simulink model "sm_vehicle_2axle_heave_roll_mu"  (R2025b)
settings: Solver=ode23t  StartTime=0.0  StopTime=14.2  MaxStep=0.2  RelTol=1e-3  AbsTol=1e-3  EnableMultiTasking=on
PostLoadFcn:
  | sm_vehicle_2axle_heave_roll_param
  | sm_vehicle_2axle_heave_roll_scene
  | sm_vehicle_2axle_heave_roll_config_maneuver(bdroot,VehicleData,'plateau');
  | set_param([bdroot '/Vehicle'],'popup_surface_conditions','Checker Right');
StartFcn:
  | tic
StopFcn:
  | Elapsed_Sim_Time = toc;
undefined symbols (not defined in the file): brake_trqTs, Disc, FL, FR, Hydraulic, InitVehicle, Mode, RL, RR, SceneData, valve_maxA, valve_maxO, VehicleData, X, Y, Z
libraries: fl_lib x92, sm_lib x43, nesl_utility x40, sm_vehicle_utilities_lib x21, sdlc_lib x8, SimscapeFluids_lib x8, simulink x2, simulink_extras x1
(part 1 of 5)
CloseFcn:
  | try,close(h1_sm_vehicle_2axle_heave_roll),end
  | clear h1_sm_vehicle_2axle_heave_roll
  | try,close(h2_sm_vehicle_2axle_heave_roll),end
  | clear h2_sm_vehicle_2axle_heave_roll
  | try,close(h3_sm_vehicle_2axle_heave_roll),end
  | clear h3_sm_vehicle_2axle_heave_roll
  | 
  | 
  | clear simlog_sm_vehicle_2axle_heave_roll
  | clear logsout_sm_vehicle_2axle_heave_roll
Description:
  | Vehicle Dynamics, 14 DOF Model, Varying Surface Friction
  | 
  | Copyright 2022-2024 The MathWorks, Inc.
settings Model: Creator=smiller  LastModifiedBy=bob
settings SolverCC: AutoScaleAbsTol=off  AlgebraicLoopSolver=TrustRegion
settings DataIOCC: SaveFormat=Array  SaveOutput=off  ReturnWorkspaceOutputs=off  SignalLoggingName=logsout_sm_vehicle_2axle_heave_roll_mu  OutputTimes=[0:0.01:10]
settings OptimizationCC: ReuseModelBlockBuffer=off  ExpressionDepthLimit=2147483647.0  LifeSpan=inf
settings DebuggingCC: UnderspecifiedInitializationDetection=Classic  MergeDetectMultiDrivingBlocksExec=none  SolverPrmCheckMsg=warning  UnconnectedInputMsg=warning  UnconnectedOutputMsg=warning  UnconnectedLineMsg=warning  StateNameClashWarn=warning  PregeneratedLibrarySubsystemCodeDiagnostic=none  SFUnexpectedBacktrackingDiag=warning  SFNoUnconditionalDefaultTransitionDiag=warning  SFExecutionAtInitializationDiag=none  ArithmeticOperatorsInVariantConditions=warning
settings HardwareCC: ProdBitPerPointer=32.0  ProdBitPerSizeT=32.0  ProdBitPerPtrDiffT=32.0  ProdLargestAtomicFloat=None  ProdIntDivRoundTo=Undefined  ProdEndianess=Unspecified  ProdWordSize=32.0  ProdHWDeviceType=32-bit Generic
settings ModelReferenceCC: EnableRefExpFcnMdlSchedulingChecks=on  PropagateSignalLabelsOutOfModel=off
settings SFSimCC: SimUseLocalCustomCode=off  CustomCodeUndefinedFunction=UseInterfaceOnly
settings RTWCC: RTWUseLocalCustomCode=off  GPUComputeCapability=3.5  DLArmComputeVersion=19.05
settings CodeAppCC: StateflowObjectComments=on
settings GRTTargetCC: TargetLangStandard=C89/C90 (ANSI)
settings ConfigComp: CovMetricSettings=dw  CovSaveCumulativeToWorkspaceVar=on  CovSaveSingleToWorkspaceVar=on  CovExternalEMLEnable=off
settings SimscapeCC: SimscapeNormalizeSystem=off  SimscapeLogType=all  SimscapeLogToSDI=on  SimscapeLogName=simlog_sm_vehicle_2axle_heave_roll_mu  SimscapeLogLimitData=off  SimscapeLogDataHistory=50000.0
settings ConfigurationSet: Description=SimMechanics 2G
settings DiagnosticsConfigSet: SimMechanicsUnconnectedFramePorts=none  SimMechanicsConflictingReferenceFrames=none
settings ExplorerConfigSet: InternalSimMechanicsExplorerSettings="<ExplorerConfiguration><canonicalview>default</canonicalview><AnimationSetting><BasePlaybackSpeed>1.0</BasePlaybackSpeed><PlaybackSpeedFactor>2.0</PlaybackSpeedFactor></AnimationSetting><TilePanel><TileInfo><Tiles Columns=\"2\" Count=\"3\" Rows=\"2\"><Column Weight=\"0.6147\"/><Column Weight=\"0.3853\"/><Row Weight=\"0.3693\"/><Row Weight=\"0.6307\"/><Tile Height=\"1\" Width=\"1\" X=\"0\" Y=\"0\"/><Tile Height=\"1\" Width=\"1\" X=\"0\" Y=\"1\"/><Tile Height=\"2\" Width=\"1\" X=\"1\" Y=\"0\"/></Tiles></TileInfo><SceneInfo><SceneViewer><BGColor><R>1</R><G>1</G><B>1</B></BGColor><Camera><DoPerspective>on</DoPerspective><Position><X>-1.49999999999999911</X><Y>1.54074395550978868e-32</Y><Z>10.6999999999999993</Z></Position><Center><X>-1.49999999999999911</X><Y>1.54074395550978868e-32</Y><Z>9.69999999999999929</Z></Center><Up><X>0</X><Y>1</Y><Z>0</Z></Up><ViewLimDist>1</ViewLimDist><YLim>0.466307658154998583</YLim><XLim>1.34838716914770518</XLim></Camera></SceneViewer><SceneViewer><BGColor><R>1</R><G>1</G><B>1</B></BGColor><Camera><DoPerspective>on</DoPerspective><Position><X>2.34000000000000163</X><Y>-3.20000000000000151</Y><Z>1.80000000000000004</Z></Position><Center><X>1.58973091910295716</X><Y>-2.57477576591913149</Y><Z>1.58507916953470085</Z></Center><Up><X>-0.16510675539218278</X><Y>0.137588962826818928</Y><Z>0.976631474319820447</Z></Up><ViewLimDist>1</ViewLimDist><YLim>0.466307658154998583</YLim><XLim>0.779836453951521791</XLim></Camera></SceneViewer><SceneViewer><BGColor><R>1</R><G>1</G><B>1</B></BGColor><Camera><DoPerspective>on</DoPerspective><Position><X>-6.5</X><Y>3.46944695195361419e-16</Y><Z>1.79999999999999982</Z></Position><Center><X>-5.52335553329491002</X><Y>3.46944695195361419e-16</Y><Z>1.58513821732488003</Z></Center><Up><X>0.214861782675119795</X><Y>-1.71056941445900502e-49</Y><Z>0.976644466705089975</Z></Up><ViewLimDist>1</ViewLimDist><YLim>0.466307658154998583</YLim><XLim>0.303969645724483983</XLim></Camera></SceneViewer></SceneInfo></TilePanel><MechEditorPanel><Cameras><Camera><Id>Camera1</Id><Value><Name>Track FixO FR</Name><NativeCamera><PositionTrackingFeature>Vehicle.Camera_Frames.Frame_FixO_FR.R</PositionTrackingFeature><CenterTrackingFeature>Vehicle.Camera_Frames.Frame_FixO_FR.R</CenterTrackingFeature><UpVectorTrackingFeature>Vehicle.Camera_Frames.Frame_FixO_FR.R</UpVectorTrackingFeature><CenterTrackingOrigin>off</CenterTrackingOrigin><CenterTrackingDirection>+X</CenterTrackingDirection><UpVectorTrackingDirection>+Z</UpVectorTrackingDirection></NativeCamera></Value></Camera><Camera><Id>Camera2</Id><Value><Name>Track FixO Right</Name><NativeCamera><PositionTrackingFeature>Vehicle.Camera_Frames.Frame_FixO_Right.R</PositionTrackingFeature><CenterTrackingFeature>Vehicle.Camera_Frames.Frame_FixO_Right.R</CenterTrackingFeature><UpVectorTrackingFeature>Vehicle.Camera_Frames.Frame_FixO_Right.R</UpVectorTrackingFeature><CenterTrackingOrigin>off</CenterTrackingOrigin><CenterTrackingDirection>+X</CenterTrackingDirection><UpVectorTrackingDirection>+Z</UpVectorTrackingDirection></NativeCamera></Value></Camera><Camera><Id>Camera3</Id><Value><Name>Track FixO RR</Name><NativeCamera><PositionTrackingFeature>Vehicle.Camera_Frames.Frame_FixO_RR.R</PositionTrackingFeature><CenterTrackingFeature>Vehicle.Camera_Frames.Frame_FixO_RR.R</CenterTrackingFeature><UpVectorTrackingFeature>Vehicle.Camera_Frames.Frame_FixO_RR.R</UpVectorTrackingFeature><CenterTrackingOrigin>off</CenterTrackingOrigin><CenterTrackingDirection>+X</CenterTrackingDirection><UpVectorTrackingDirection>+Z</UpVectorTrackingDirection></NativeCamera></Value></Camera><Camera><Id>Camera4</Id><Value><Name>Track FixO RL</Name><NativeCamera><PositionTrackingFeature>Vehicle.Camera_Frames.Frame_FixO_RL.R</PositionTrackingFeature><CenterTrackingFeature>Vehicle.Camera_Frames.Frame_FixO_RL.R</CenterTrackingFeature><UpVectorTrackingFeature>Vehicle.Camera_Frames.Frame_FixO_RL.R</UpVectorTrackingFeature><CenterTrackingOrigin>off</CenterTrackingOrigin><CenterTrackingDirection>+X</CenterTrackingDirection><UpVectorTrackingDirection>+Z</UpVectorTrackingDirection></NativeCamera></Value></Camera><Camera><Id>Camera5</Id><Value><Name>Track FixO Left</Name><NativeCamera><PositionTrackingFeature>Vehicle.Camera_Frames.Frame_FixO_Left.R</PositionTrackingFeature><CenterTrackingFeature>Vehicle.Camera_Frames.Frame_FixO_Left.R</CenterTrackingFeature><UpVectorTrackingFeature>Vehicle.Camera_Frames.Frame_FixO_Left.R</UpVectorTrackingFeature><CenterTrackingOrigin>off</CenterTrackingOrigin><CenterTrackingDirection>+X</CenterTrackingDirection><UpVectorTrackingDirection>+Z</UpVectorTrackingDirection></NativeCamera></Value></Camera><Camera><Id>Camera6</Id><Value><Name>Track FixO FL</Name><NativeCamera><PositionTrackingFeature>Vehicle.Camera_Frames.Frame_FixO_FL.R</PositionTrackingFeature><CenterTrackingFeature>Vehicle.Camera_Frames.Frame_FixO_FL.R</CenterTrackingFeature><UpVectorTrackingFeature>Vehicle.Camera_Frames.Frame_FixO_FL.R</UpVectorTrackingFeature><CenterTrackingOrigin>off</CenterTrackingOrigin><CenterTrackingDirection>+X</CenterTrackingDirection><UpVectorTrackingDirection>+Z</UpVectorTrackingDirection></NativeCamera></Value></Camera><Camera><Id>Camera7</Id><Value><Name>Track FixO Top</Name><NativeCamera><PositionTrackingFeature>Vehicle.Camera_Frames.Frame_FixO_Top.R</PositionTrackingFeature><CenterTrackingFeature>Vehicle.Camera_Frames.Frame_FixO_Top.R</CenterTrackingFeature><UpVectorTrackingFeature>Vehicle.Camera_Frames.Frame_FixO_Top.R</UpVectorTrackingFeature><CenterTrackingOrigin>off</CenterTrackingOrigin><CenterTrackingDirection>+X</CenterTrackingDirection><UpVectorTrackingDirection>+Z</UpVectorTrackingDirection></NativeCamera></Value></Camera><Camera><Id>Camera8</Id><Value><Name>Track FixO Front</Name><NativeCamera><PositionTrackingFeature>Vehicle.Camera_Frames.Frame_FixO_Front.R</PositionTrackingFeature><CenterTrackingFeature>Vehicle.Camera_Frames.Frame_FixO_Front.R</CenterTrackingFeature><UpVectorTrackingFeature>Vehicle.Camera_Frames.Frame_FixO_Front.R</UpVectorTrackingFeature><CenterTrackingOrigin>off</CenterTrackingOrigin><CenterTrackingDirection>+X</CenterTrackingDirection><UpVectorTrackingDirection>+Z</UpVectorTrackingDirection></NativeCamera></Value></Camera><Camera><Id>Camera9</Id><Value><Name>Track FixO Rear</Name><NativeCamera><PositionTrackingFeature>Vehicle.Camera_Frames.Frame_FixO_Rear.R</PositionTrackingFeature><CenterTrackingFeature>Vehicle.Camera_Frames.Frame_FixO_Rear.R</CenterTrackingFeature><UpVectorTrackingFeature>Vehicle.Camera_Frames.Frame_FixO_Rear.R</UpVectorTrackingFeature><CenterTrackingOrigin>off</CenterTrackingOrigin><CenterTrackingDirection>+X</CenterTrackingDirection><UpVectorTrackingDirection>+Z</UpVectorTrackingDirection></NativeCamera></Value></Camera><Camera><Id>Camera10</Id><Value><Name>Track FR</Name><NativeCamera><PositionTrackingFeature>Vehicle.Camera_Frames.Frame_FR.R</PositionTrackingFeature><CenterTrackingFeature>Vehicle.Camera_Frames.Frame_FR.R</CenterTrackingFeature><UpVectorTrackingFeature>Vehicle.Camera_Frames.Frame_FR.R</UpVectorTrackingFeature><CenterTrackingOrigin>off</CenterTrackingOrigin><CenterTrackingDirection>+X</CenterTrackingDirection><UpVectorTrackingDirection>+Z</UpVectorTrackingDirection></NativeCamera></Value></Camera><Camera><Id>Camera11</Id><Value><Name>Track Right</Name><NativeCamera><PositionTrackingFeature>Vehicle.Camera_Frames.Frame_Right.R</PositionTrackingFeature><CenterTrackingFeature>Vehicle.Camera_Frames.Frame_Right.R</CenterTrackingFeature><UpVectorTrackingFeature>Vehicle.Camera_Frames.Frame_Right.R</UpVectorTrackingFeature><CenterTrackingOrigin>off</CenterTrackingOrigin><CenterTrackingDirection>+X</CenterTrackingDirection><UpVectorTrackingDirection>+Z</UpVectorTrackingDirection></NativeCamera></Value></Camera><Camera><Id>Camera12</Id><Value><Name>Track RR</Name><NativeCamera><PositionTrackingFeature>Vehicle.Camera_Frames.Frame_RR.R</PositionTrackingFeature><CenterTrackingFeature>Vehicle.Camera_Frames.Frame_RR.R</CenterTrackingFeature><UpVectorTrackingFeature>Vehicle.Camera_Frames.Frame_RR.R</UpVectorTrackingFeature><CenterTrackingOrigin>off</CenterTrackingOrigin><CenterTrackingDirection>+X</CenterTrackingDirection><UpVectorTrackingDirection>+Z</UpVectorTrackingDirection></NativeCamera></Value></Camera><Camera><Id>Camera13</Id><Value><Name>Track RL</Name><NativeCamera><PositionTrackingFeature>Vehicle.Camera_Frames.Frame_RL.R</PositionTrackingFeature><CenterTrackingFeature>Vehicle.Camera_Frames.Frame_RL.R</CenterTrackingFeature><UpVectorTrackingFeature>Vehicle.Camera_Frames.Frame_RL.R</UpVectorTrackingFeature><CenterTrackingOrigin>off</CenterTrackingOrigin><CenterTrackingDirection>+X</CenterTrackingDirection><UpVectorTrackingDirection>+Z</UpVectorTrackingDirection></NativeCamera></Value></Camera><Camera><Id>Camera14</Id><Value><Name>Track Left</Name><NativeCamera><PositionTrackingFeature>Vehicle.Camera_Frames.Frame_Left.R</PositionTrackingFeature><CenterTrackingFeature>Vehicle.Camera_Frames.Frame_Left.R</CenterTrackingFeature><UpVectorTrackingFeature>Vehicle.Camera_Frames.Frame_Left.R</UpVectorTrackingFeature><CenterTrackingOrigin>off</CenterTrackingOrigin><CenterTrackingDirection>+X</CenterTrackingDirection><UpVectorTrackingDirection>+Z</UpVectorTrackingDirection></NativeCamera></Value></Camera><Camera><Id>Camera15</Id><Value><Name>Track FL</Name><NativeCamera><PositionTrackingFeature>Vehicle.Camera_Frames.Frame_FL.R</PositionTrackingFeature><CenterTrackingFeature>Vehicle.Camera_Frames.Frame_FL.R</CenterTrackingFeature><UpVectorTrackingFeature>Vehicle.Camera_Frames.Frame_FL.R</UpVectorTrackingFeature><CenterTrackingOrigin>off</CenterTrackingOrigin><CenterTrackingDirection>+X</CenterTrackingDirection><UpVectorTrackingDirection>+Z</UpVectorTrackingDirection></NativeCamera></Value></Camera><Camera><Id>Camera16</Id><Value><Name>Track Top</Name><NativeCamera><PositionTrackingFeature>Vehicle.Camera_Frames.Frame_Top.R</PositionTrackingFeature><CenterTrackingFeature>Vehicle.Camera_Frames.Frame_Top.R</CenterTrackingFeature><UpVectorTrackingFeature>Vehicle.Camera_Frames.Frame_Top.R</UpVectorTrackingFeature><CenterTrackingOrigin>off</CenterTrackingOrigin><CenterTrackingDirection>+X</CenterTrackingDirection><UpVectorTrackingDirection>+Z</UpVectorTrackingDirection></NativeCamera></Value></Camera><Camera><Id>Camera17</Id><Value><Name>Track Front</Name><NativeCamera><PositionTrackingFeature>Vehicle.Camera_Frames.Frame_Front.R</PositionTrackingFeature><CenterTrackingFeature>Vehicle.Camera_Frames.Frame_Front.R</CenterTrackingFeature><UpVectorTrackingFeature>Vehicle.Camera_Frames.Frame_Front.R</UpVectorTrackingFeature><CenterTrackingOrigin>off</CenterTrackingOrigin><CenterTrackingDirection>+X</CenterTrackingDirection><UpVectorTrackingDirection>+Z</UpVectorTrackingDirection></NativeCamera></Value></Camera><Camera><Id>Camera18</Id><Value><Name>Track Rear</Name><NativeCamera><PositionTrackingFeature>Vehicle.Camera_Frames.Frame_Rear.R</PositionTrackingFeature><CenterTrackingFeature>Vehicle.Camera_Frames.Frame_Rear.R</CenterTrackingFeature><UpVectorTrackingFeature>Vehicle.Camera_Frames.Frame_Rear.R</UpVectorTrackingFeature><CenterTrackingOrigin>off</CenterTrackingOrigin><CenterTrackingDirection>+X</CenterTrackingDirection><UpVectorTrackingDirection>+Z</UpVectorTrackingDirection></NativeCamera></Value></Camera><Camera><Id>Camera19</Id><Value><Name>Track SuspF</Name><NativeCamera><PositionTrackingFeature>Vehicle.Camera_Frames.Frame_SuspF.R</PositionTrackingFeature><CenterTrackingFeature>Vehicle.Camera_Frames.Frame_SuspF.R</CenterTrackingFeature><UpVectorTrackingFeature>Vehicle.Camera_Frames.Frame_SuspF.R</UpVectorTrackingFeature><CenterTrackingOrigin>off</CenterTrackingOrigin><CenterTrackingDirection>+X</CenterTrackingDirection><UpVectorTrackingDirection>+Z</UpVectorTrackingDirection></NativeCamera></Value></Camera><Camera><Id>Camera20</Id><Value><Name>Track SuspR</Name><NativeCamera><PositionTrackingFeature>Vehicle.Camera_Frames.Frame_SuspR.R</PositionTrackingFeature><CenterTrackingFeature>Vehicle.Camera_Frames.Frame_SuspR.R</CenterTrackingFeature><UpVectorTrackingFeature>Vehicle.Camera_Frames.Frame_SuspR.R</UpVectorTrackingFeature><CenterTrackingOrigin>off</CenterTrackingOrigin><CenterTrackingDirection>+X</CenterTrackingDirection><UpVectorTrackingDirection>+Z</UpVectorTrackingDirection></NativeCamera></Value></Camera><Camera><Id>Camera21</Id><Value><Name>Track WheelFR</Name><NativeCamera><PositionTrackingFeature>Vehicle.Camera_Frames.Frame_Wheel_FR.R</PositionTrackingFeature><CenterTrackingFeature>Vehicle.Camera_Frames.Frame_Wheel_FR.R</CenterTrackingFeature><UpVectorTrackingFeature>Vehicle.Camera_Frames.Frame_Wheel_FR.R</UpVectorTrackingFeature><CenterTrackingOrigin>off</CenterTrackingOrigin><CenterTrackingDirection>+X</CenterTrackingDirection><UpVectorTrackingDirection>+Z</UpVectorTrackingDirection></NativeCamera></Value></Camera><Camera><Id>Camera22</Id><Value><Name>Track WheelRR</Name><NativeCamera><PositionTrackingFeature>Vehicle.Camera_Frames.Frame_Wheel_RR.R</PositionTrackingFeature><CenterTrackingFeature>Vehicle.Camera_Frames.Frame_Wheel_RR.R</CenterTrackingFeature><UpVectorTrackingFeature>Vehicle.Camera_Frames.Frame_Wheel_RR.R</UpVectorTrackingFeature><CenterTrackingOrigin>off</CenterTrackingOrigin><CenterTrackingDirection>+X</CenterTrackingDirection><UpVectorTrackingDirection>+Z</UpVectorTrackingDirection></NativeCamera></Value></Camera><Camera><Id>Camera23</Id><Value><Name>Track WheelRL</Name><NativeCamera><PositionTrackingFeature>Vehicle.Camera_Frames.Frame_Wheel_RL.R</PositionTrackingFeature><CenterTrackingFeature>Vehicle.Camera_Frames.Frame_Wheel_RL.R</CenterTrackingFeature><UpVectorTrackingFeature>Vehicle.Camera_Frames.Frame_Wheel_RL.R</UpVectorTrackingFeature><CenterTrackingOrigin>off</CenterTrackingOrigin><CenterTrackingDirection>+X</CenterTrackingDirection><UpVectorTrackingDirection>+Z</UpVectorTrackingDirection></NativeCamera></Value></Camera><Camera><Id>Camera24</Id><Value><Name>Track WheelFL</Name><NativeCamera><PositionTrackingFeature>Vehicle.Camera_Frames.Frame_Wheel_FL.R</PositionTrackingFeature><CenterTrackingFeature>Vehicle.Camera_Frames.Frame_Wheel_FL.R</CenterTrackingFeature><UpVectorTrackingFeature>Vehicle.Camera_Frames.Frame_Wheel_FL.R</UpVectorTrackingFeature><CenterTrackingOrigin>off</CenterTrackingOrigin><CenterTrackingDirection>+X</CenterTrackingDirection><UpVectorTrackingDirection>+Z</UpVectorTrackingDirection></NativeCamera></Value></Camera><Camera><Id>Camera25</Id><Value><Name>View Seat FL</Name><NativeCamera><PositionTrackingFeature>Vehicle.Camera_Frames.Frame_View_Seat_FL.R</PositionTrackingFeature><CenterTrackingFeature>Vehicle.Camera_Frames.Frame_View_Seat_FL.R</CenterTrackingFeature><UpVectorTrackingFeature>Vehicle.Camera_Frames.Frame_View_Seat_FL.R</UpVectorTrackingFeature><CenterTrackingOrigin>off</CenterTrackingOrigin><CenterTrackingDirection>+X</CenterTrackingDirection><UpVectorTrackingDirection>+Z</UpVectorTrackingDirection></NativeCamera></Value></Camera><Camera><Id>Camera26</Id><Value><Name>View Seat FR</Name><NativeCamera><PositionTrackingFeature>Vehicle.Camera_Frames.Frame_View_Seat_FR.R</PositionTrackingFeature><CenterTrackingFeature>Vehicle.Camera_Frames.Frame_View_Seat_FR.R</CenterTrackingFeature><UpVectorTrackingFeature>Vehicle.Camera_Frames.Frame_View_Seat_FR.R</UpVectorTrackingFeature><CenterTrackingOrigin>off</CenterTrackingOrigin><CenterTrackingDirection>+X</CenterTrackingDirection><UpVectorTrackingDirection>+Z</UpVectorTrackingDirection></NativeCamera></Value></Camera><Camera><Id>Camera27</Id><Value><Name>View Susp FR</Name><NativeCamera><PositionTrackingFeature>Vehicle.Camera_Frames.Frame_View_Susp_FR.R</PositionTrackingFeature><CenterTrackingFeature>Vehicle.Camera_Frames.Frame_View_Susp_FR.R</CenterTrackingFeature><UpVectorTrackingFeature>Vehicle.Camera_Frames.Frame_View_Susp_FR.R</UpVectorTrackingFeature><CenterTrackingOrigin>off</CenterTrackingOrigin><CenterTrackingDirection>+X</CenterTrackingDirection><UpVectorTrackingDirection>+Z</UpVectorTrackingDirection></NativeCamera></Value></Camera><Camera><Id>Camera28</Id><Value><Name>View Susp RR</Name><NativeCamera><PositionTrackingFeature>Vehicle.Camera_Frames.Frame_View_Susp_RR.R</PositionTrackingFeature><CenterTrackingFeature>Vehicle.Camera_Frames.Frame_View_Susp_RR.R</CenterTrackingFeature><UpVectorTrackingFeature>Vehicle.Camera_Frames.Frame_View_Susp_RR.R</UpVectorTrackingFeature><CenterTrackingOrigin>off</CenterTrackingOrigin><CenterTrackingDirection>+X</CenterTrackingDirection><UpVectorTrackingDirection>+Z</UpVectorTrackingDirection></NativeCamera></Value></Camera><Camera><Id>Camera29</Id><Value><Name>View Susp RL</Name><NativeCamera><PositionTrackingFeature>Vehicle.Camera_Frames.Frame_View_Susp_RL.R</PositionTrackingFeature><CenterTrackingFeature>Vehicle.Camera_Frames.Frame_View_Susp_RL.R</CenterTrackingFeature><UpVectorTrackingFeature>Vehicle.Camera_Frames.Frame_View_Susp_RL.R</UpVectorTrackingFeature><CenterTrackingOrigin>off</CenterTrackingOrigin><CenterTrackingDirection>+X</CenterTrackingDirection><UpVectorTrackingDirection>+Z</UpVectorTrackingDirection></NativeCamera></Value></Camera><Camera><Id>Camera30</Id><Value><Name>View Susp FL</Name><NativeCamera><PositionTrackingFeature>Vehicle.Camera_Frames.Frame_View_Susp_FL.R</PositionTrackingFeature><CenterTrackingFeature>Vehicle.Camera_Frames.Frame_View_Susp_FL.R</CenterTrackingFeature><UpVectorTrackingFeature>Vehicle.Camera_Frames.Frame_View_Susp_FL.R</UpVectorTrackingFeature><CenterTrackingOrigin>off</CenterTrackingOrigin><CenterTrackingDirection>+X</CenterTrackingDirection><UpVectorTrackingDirection>+Z</UpVectorTrackingDirection></NativeCamera></Value></Camera><Camera><Id>Camera31</Id><Value><Name>Dolly Camera</Name><NativeCamera><PositionTrackingFeature>Vehicle.Camera_Frames.Frame_Dolly.R</PositionTrackingFeature><CenterTrackingFeature>Vehicle.Camera_Frames.Frame_Dolly.R</CenterTrackingFeature><UpVectorTrackingFeature>Vehicle.Camera_Frames.Frame_Dolly.R</UpVectorTrackingFeature><CenterTrackingOrigin>off</CenterTrackingOrigin><CenterTrackingDirection>+X</CenterTrackingDirection><UpVectorTrackingDirection>+Z</UpVectorTrackingDirection></NativeCamera></Value></Camera><Camera><Id>Camera32</Id><Value><Name>Track Dolly Camera</Name><NativeCamera><PositionTrackingFeature>Vehicle.Camera_Frames.Frame_Dolly.R</PositionTrackingFeature><CenterTrackingFeature>Vehicle.Camera_Frames.Transform_Camera_Ref.F</CenterTrackingFeature><UpVectorTrackingFeature>Vehicle.Camera_Frames.World_Frame.W</UpVectorTrackingFeature><CenterTrackingOrigin>on</CenterTrackingOrigin><UpVectorTrackingDirection>+Z</UpVectorTrackingDirection></NativeCamera></Value></Camera></Cameras><GfxPanelCameraMap><MapElement CameraMLId=\"Camera7\" GfxPanelIndex=\"0\"/><MapElement CameraMLId=\"Camera1\" GfxPanelIndex=\"1\"/><MapElement CameraMLId=\"Camera9\" GfxPanelIndex=\"2\"/></GfxPanelCameraMap><VideoCreator><PlaybackSpeedRatio>1.0</PlaybackSpeedRatio><FrameRate>30</FrameRate><VideoFormat>MPEG-4</VideoFormat><FrameSize>[800 450]</FrameSize></VideoCreator></MechEditorPanel></ExplorerConfiguration>"

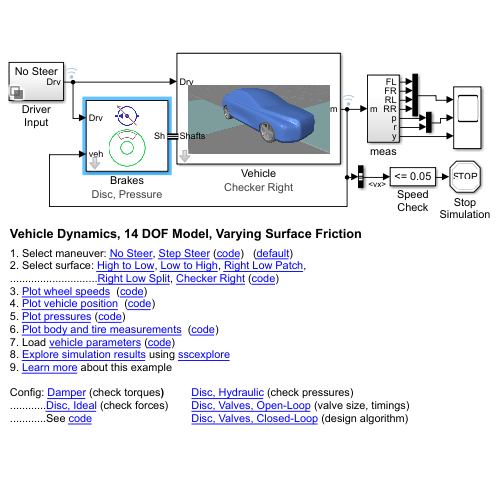
[thumbnail: Simulink's stored preview of the top-level diagram]
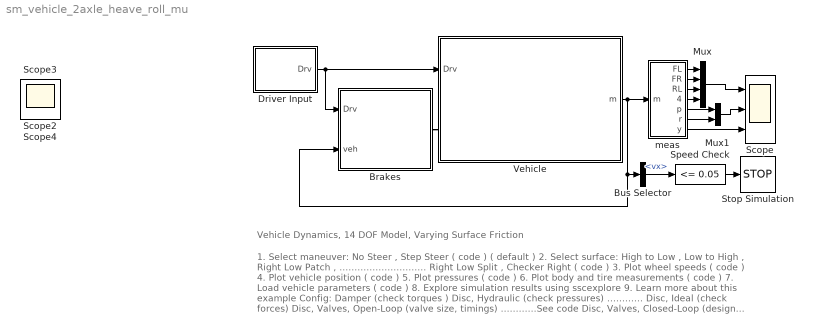
== system sm_vehicle_2axle_heave_roll_mu ==
  note: Vehicle Dynamics, 14 DOF Model, Varying Surface Friction
  note: 1. Select maneuver: No Steer , Step Steer ( code ) ( default )
      | 2. Select surface: High to Low , Low to High , Right Low Patch ,
      | ............................. Right Low Split , Checker Right ( code )
      | 3. Plot wheel speeds ( code )
      | 4. Plot vehicle position ( code )
      | 5. Plot pressures ( code )
      | 6. Plot body and tire measurements ( code )
      | 7. Load vehicle parameters ( code )
      | 8. Explore simulation results using sscexplore
      | 9. Learn more about this example
      |
      | Config: Damper (check torques ) Disc, Hydraulic (check pressures)
      | ............ Disc, Ideal (check forces) Disc, Valves, Open-Loop (valve size, timings)
      | ............See code Disc, Valves, Closed-Loop (design algorithm)
  Brakes : Subsystem  mask(Braking Model){brake_model=Disc, Hydraulic Pressure   (estimate required caliper pressure), control_mode=Mode, brake_type=Disc, actuator_type=Hydraulic}
      mask prompts: brake_model "Select Brake Model"; control_mode "Control Mode"; brake_type "Braking System"; actuator_type "Actuator Type"
      mask help: Select braking model type. The options below configure the braking model to permit focus on a specific aspect of the design.
      mask init:
      | if(brake_type==1)
      |     set_param(gcb,'LabelModeActiveChoice','Damper');
      |     % Variant not used, but set for Block Annotation
      |     set_param(gcb,'actuator_type','Ideal');
      | elseif(brake_type==2)
      |     set_param(gcb,'LabelModeActiveChoice','Disc');
      | end
      settings: AttributesFormatString=Disc, Pressure
      mask TypeOptions brake_model: Damper                           (estimate required brake torque) | Disc, Ideal                       (estimate required caliper force) | Disc, Hydraulic Pressure   (estimate required caliper pressure) | Disc, Valves, Open-Loop   (refine valve requirements) | Disc, Valves, Closed-Loop (design control algorithm)
      mask Callback brake_model:
      | maskObj = Simulink.Mask.get(gcb);
      | bkm_h = maskObj.getParameter('brake_model');
      | brm_index = find(strcmp(bkm_h.Value,bkm_h.TypeOptions));
      | sm_vehicle_2axle_heave_roll_mu_config_abs_system(gcb,brm_index);
      mask TypeOptions control_mode: Brake Control/control_mode
      mask TypeOptions brake_type: Brakes/brake_type
      mask TypeOptions actuator_type: Brakes/actuator_type
      mask Display:
      | actuator_type = get_param(gcb,'actuator_type');
      | control_mode = get_param(gcb,'control_mode');
      | brake_type = get_param(gcb,'brake_type');
      | 
      | if(strcmpi(brake_type,'damper'))
      | image('sm_vehicle_2axle_brake_damper.png');
      | elseif(strcmpi(actuator_type,'ideal'))
      | image('sm_vehicle_2axle_brake_disc_ideal.png');
      | elseif(strcmpi(actuator_type,'hydraulic'))
      | image('sm_vehicle_2axle_brake_disc_hydraulic.png');
      | elseif(strcmpi(control_mode,'valve closed-loop'))
      | image('sm_vehicle_2axle_brake_disc_valves_ctrl.png');
      | else
      | image('sm_vehicle_2axle_brake_disc_valves.png');
      | end
  Bus Selector : BusSelector  OutputSignals=Body.vx
  Driver Input : Subsystem  Variant=on  VariantControlMode=label  LabelModeActiveChoice=NoSteer
  Mux : Mux
  Mux1 : Mux  Inputs=2
  Scope : Scope  NumInputPorts=3
      settings: ActiveDisplayYMinimum=-7.08357  ActiveDisplayYMaximum=66.13125
  Speed Check : simulink/Logic and Bit Operations/Compare To Constant  relop=<=  const=0.05  OutDataTypeStr=boolean
  Stop Simulation : Stop
  Vehicle : Subsystem  mask(Vehicle and Scene){vehdata=VehicleData, initveh=InitVehicle, popup_surface_conditions=Checker Right}
      mask prompts: vehdata "Vehicle Data (structure)"; initveh "Initial Position, Velocity (structure)"; popup_surface_conditions "Surface Conditions"
      mask help: Models a vehicle with a configurable scene. Vehicle parameters are defined within a single data structure. A separate data structure defines the initial position, orientation, and speed of the vehicle and the wheels.
      mask init:
      | surface_name = lower(strrep(get_param(gcb,'popup_surface_conditions'),' ','_'));
      | 
      | [mu_surface, p1, p2] = sm_vehicle_2axle_heave_roll_mu_config_icepatch(surface_name);
      settings: AttributesFormatString=%<popup_surface_conditions>
      mask TypeOptions popup_surface_conditions: High to Low | Low to High | Right Low Patch | Right Low Split | Checker Right
      mask Display:
      | surface_name = lower(strrep(get_param(gcb,'popup_surface_conditions'),' ','_'));
      | 
      | image(['sm_vehicle_2axle_heave_roll_vehicle_mu_' surface_name '.png']);
  meas : Subsystem
  Scope2 : Scope
      settings: DataLoggingMaxPoints=7500  DataLoggingSaveFormat=Array
  Scope3 : Scope
      settings: DataLoggingMaxPoints=7500  DataLoggingSaveFormat=Array
  Scope4 : Scope
      settings: DataLoggingMaxPoints=7500  DataLoggingVariableName=ScopeData2  DataLoggingSaveFormat=Array
  wires:
  Driver Input/1(Drv) -> Vehicle/1(Drv), Brakes/1(Drv)
  Vehicle/1(m) -> meas/1(m), Bus Selector/1, Brakes/2(veh)
  Mux/1 -> Scope/1
  meas/1(FL) -> Mux/1
  meas/2(FR) -> Mux/2
  meas/3(RL) -> Mux/3
  meas/4(RR) -> Mux/4
  meas/5(p) -> Mux1/1
  meas/6(r) -> Mux1/2
  Mux1/1 -> Scope/2
  meas/7(y) -> Scope/3
  Speed Check/1 -> Stop Simulation/1
  Bus Selector/1 -> Speed Check/1  "<vx>"
  connections:
  Brakes/RConn1 -- Vehicle/LConn1

== system sm_vehicle_2axle_heave_roll_mu/Brakes ==
  Drv : Inport
  BusElementIn1 : Inport  Port=2  PortName=veh
  Brake Control : Subsystem  Variant=on  VariantControlMode=label  VariantControl=Variant1  LabelModeActiveChoice=Mode  mask(Brake Control){control_mode=Mode}
      mask prompts: control_mode "Control Mode"
      mask help: Braking control system. Can set mode (Apply, Hold, Release) or states of apply and release valves.
      mask init:
      | if(control_mode==1)
      |     set_param(gcb,'LabelModeActiveChoice','Mode');
      | elseif(control_mode==2)
      |     set_param(gcb,'LabelModeActiveChoice','Valve_Open_Loop');
      | elseif(control_mode==3)
      |     set_param(gcb,'LabelModeActiveChoice','Valve_Closed_Loop');
      | end
      settings: AttributesFormatString=%<control_mode>
      mask TypeOptions control_mode: Mode | Valve Open-Loop | Valve Closed-Loop
      mask Display: disp(' ')
  Brakes : Subsystem  Variant=on  VariantControlMode=label  VariantControl=Variant1  LabelModeActiveChoice=Disc  mask(Braking System){brake_type=Disc, actuator_type=Hydraulic}
      mask prompts: brake_type "Braking System"; actuator_type "Actuator Type"
      mask help: Braking actuators and hardware. Abstract variants for component sizing and valve variants for testing control algorithm.
      mask init:
      | if(brake_type==1)
      |     set_param(gcb,'LabelModeActiveChoice','Damper');
      | else
      |     set_param(gcb,'LabelModeActiveChoice','Disc');
      | end
      settings: AttributesFormatString=%<brake_type>, %<actuator_type>
      mask TypeOptions brake_type: Damper | Disc
      mask Callback brake_type:
      | maskObj = Simulink.Mask.get(gcb);
      | bkt_h = maskObj.getParameter('brake_type');
      | act_h = maskObj.getParameter('actuator_type');
      | if strcmp(get_param(gcb,'brake_type'),'Damper')
      |     act_h.Visible = 'off';
      | else
      |     act_h.Visible = 'on';
      | end
      | clear maskObj act_h bkt_h
      mask TypeOptions actuator_type: Disc/actuator_type
      mask Display:
      | blk = sm_vehicle_2axle_heave_roll_activeVariantBlock(gcb);
      | eval(get_param(blk, 'MaskDisplay'));
  Bus Selector : BusSelector  OutputSignals=BrkPedal
  Get Pressure : Subsystem
  Pressures : Scope  NumInputPorts=4
      settings: ActiveDisplayYMinimum=-217.5567  ActiveDisplayYMaximum=1958.00947
  Simscape Bus : SimscapeBus  HierarchyStrings=FR;RR;RL;FL
  Subsystem : Subsystem
  Terminator : Terminator
  Sh : PMIOPort  Side=Right
  wires:
  Brake Control/1(" Valves") -> Brakes/1(Valve)
  BusElementIn1/1 -> Subsystem/1(I)
  Drv/1 -> Bus Selector/1
  Bus Selector/1 -> Brakes/2(BrkOn)  "<BrkPedal>"
  Subsystem/1(O) -> Brake Control/1(Sensor)
  Get Pressure/3(RL) -> Pressures/3
  Get Pressure/1(FL) -> Pressures/1
  Get Pressure/4(RR) -> Pressures/4
  Get Pressure/2(FR) -> Pressures/2
  Brakes/1(" meas") -> Terminator/1, Get Pressure/1(m)  "BrkBus"
  connections:
  Brakes/RConn1 -- Simscape Bus/LConn1
  Simscape Bus/RConn1 -- Sh/RConn1
  Brakes/LConn1 -- Simscape Bus/LConn4
  Brakes/LConn2 -- Simscape Bus/LConn3
  Brakes/RConn2 -- Simscape Bus/LConn2

== system sm_vehicle_2axle_heave_roll_mu/Driver Input ==
  No Steer : Subsystem  VariantControl=NoSteer
  Step Steer : Subsystem  VariantControl=StepSteer
  Drv : Outport
